simulink model "Traj_track_mec_MAS"  (R2024b)
settings: Solver=ode3  StartTime=0.0  StopTime=300  FixedStep=0.1  RelTol=1e-3
libraries: slpidlib x8
settings Model: Creator=my  LastModifiedBy=my
settings DebuggingCC: AlgebraicLoopMsg=none

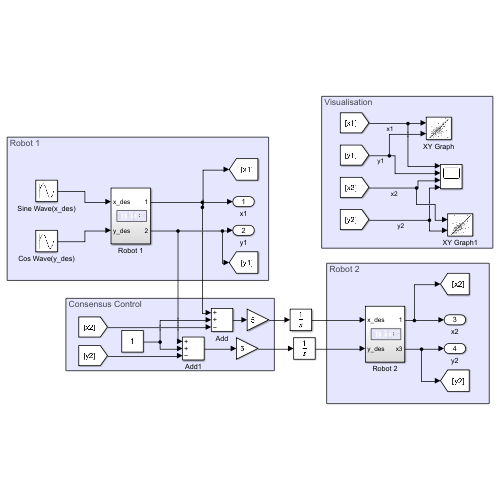
[thumbnail: Simulink's stored preview of the top-level diagram]
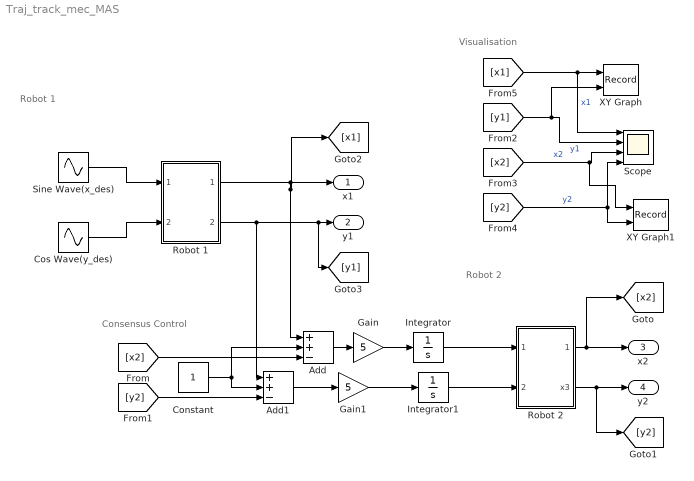
== system Traj_track_mec_MAS ==
  note: Visualisation
  note: Robot 2
  note: Robot 1
  note: Consensus Control
  Add : Sum  Inputs=++-
  Add1 : Sum  Inputs=++-
  Constant : Constant
  Cos Wave(y_des) : Sin  Frequency=0.1  Phase=pi/2  SampleTime=0
  Gain : Gain  Gain=5
  Gain1 : Gain  Gain=5
  Integrator : Integrator
  Integrator1 : Integrator
  Robot 1 : Subsystem
  Robot 2 : Subsystem
  Scope : Scope  NumInputPorts=4
  Sine Wave(x_des) : Sin  Frequency=0.1  SampleTime=0
  XY Graph : Record  FileSettingsInternal="{\"entries\":[{\"content\":{\"excelSettings\":{\"content\":{},\"type\":\"Streamout.ExcelSettings\"}},\"type\":\"Streamout.FileSettingStorage\",\"uuid\":\"\"}],\"packageUris\":[\"http:\\/\\/schema.mathworks.com\\/mf0\\/streamout_blocks\\/R2020a\"],\"version\":\"1.0\"}"  Layout=[1 1]  SignalsInternal="{\"entries\":[{\"content\":{\"signals\":[{\"content\":{\"blockPath\":[],\"dimensions\":[1],\"domain\":\"\",\"lineColor\":\"#a2142f\",\"plots\":[ 1 ],\"port\":1,\"sid\":[\"\"],\"signalID\":1,\"signalName\":\"x1\"},\"type\":\"RecordBlkView.Signal\",\"uuid\":\"\"},{\"content\":{\"blockPath\":[],\"dimensions\":[1],\"domain\":\"\",\"lineColor\":\"#139fff\",\"plots\":[ 1 ],\"port\":2,\"sid\":[\"\"],\"signalID\":2,\"signalName\":\"y1\"},\"type\":\"RecordBlkView.Signal\",\"uuid\":\"\"}]},\"type\":\"RecordBlkView.InputSignals\",\"uuid\":\"\"}],\"packageUris\":[\"http:\\/\\/schema.mathworks.com\\/mf0\\/streamout_blocks\\/R2020a\"],\"version\":\"1.0\"}"  VisualizationBindings="{\"xyplotplugin\":{\"info\":[{\"series\":[{\"bindingParametersList\":[{\"parameter\":\"X-Axis\",\"signalID\":1,\"signalName\":\"x1\"},{\"parameter\":\"Y-Axis\",\"signalID\":2,\"signalName\":\"y1\"}],\"seriesID\":0}],\"subplotID\":1}]}}"  CompatibilityTag=XY
  XY Graph1 : Record  FileSettingsInternal="{\"entries\":[{\"content\":{\"excelSettings\":{\"content\":{},\"type\":\"Streamout.ExcelSettings\"}},\"type\":\"Streamout.FileSettingStorage\",\"uuid\":\"\"}],\"packageUris\":[\"http:\\/\\/schema.mathworks.com\\/mf0\\/streamout_blocks\\/R2020a\"],\"version\":\"1.0\"}"  Layout=[1 1]  SignalsInternal="{\"entries\":[{\"content\":{\"signals\":[{\"content\":{\"blockPath\":[],\"dimensions\":[1],\"domain\":\"\",\"lineColor\":\"#a2142f\",\"plots\":[ 1 ],\"port\":1,\"sid\":[\"\"],\"signalID\":1,\"signalName\":\"x2\"},\"type\":\"RecordBlkView.Signal\",\"uuid\":\"\"},{\"content\":{\"blockPath\":[],\"dimensions\":[1],\"domain\":\"\",\"lineColor\":\"#139fff\",\"plots\":[ 1 ],\"port\":2,\"sid\":[\"\"],\"signalID\":2,\"signalName\":\"y2\"},\"type\":\"RecordBlkView.Signal\",\"uuid\":\"\"}]},\"type\":\"RecordBlkView.InputSignals\",\"uuid\":\"\"}],\"packageUris\":[\"http:\\/\\/schema.mathworks.com\\/mf0\\/streamout_blocks\\/R2020a\"],\"version\":\"1.0\"}"  VisualizationBindings="{\"xyplotplugin\":{\"info\":[{\"series\":[{\"bindingParametersList\":[{\"parameter\":\"X-Axis\",\"signalID\":1,\"signalName\":\"x2\"},{\"parameter\":\"Y-Axis\",\"signalID\":2,\"signalName\":\"y2\"}],\"seriesID\":0}],\"subplotID\":1}]}}"  CompatibilityTag=XY
  x1 : Outport
  y1 : Outport  Port=2
  x2 : Outport  Port=3
  y2 : Outport  Port=4
  wires:
  Sine Wave(x_des)/1 -> Robot 1/1(x_des)
  Cos Wave(y_des)/1 -> Robot 1/2(y_des)
  Robot 1/2(Out2) -> Add1/1, [y1], y1/1
  Robot 2/1(Out1) -> [x2], x2/1
  Robot 2/2(x3) -> [y2], y2/1
  Add/1 -> Gain/1
  Add1/1 -> Gain1/1
  Robot 1/1(Out1) -> [x1], Add/1, x1/1
  [x1] -> XY Graph/1, Scope/1  "x1"
  [y1] -> XY Graph/2, Scope/2  "y1"
  [x2] -> XY Graph1/1, Scope/3  "x2"
  [y2] -> XY Graph1/2, Scope/4  "y2"
  [x2] -> Add/3
  [y2] -> Add1/3
  Constant/1 -> Add/2, Add1/2
  Gain/1 -> Integrator/1
  Integrator/1 -> Robot 2/1(x_des)
  Gain1/1 -> Integrator1/1
  Integrator1/1 -> Robot 2/2(y_des)

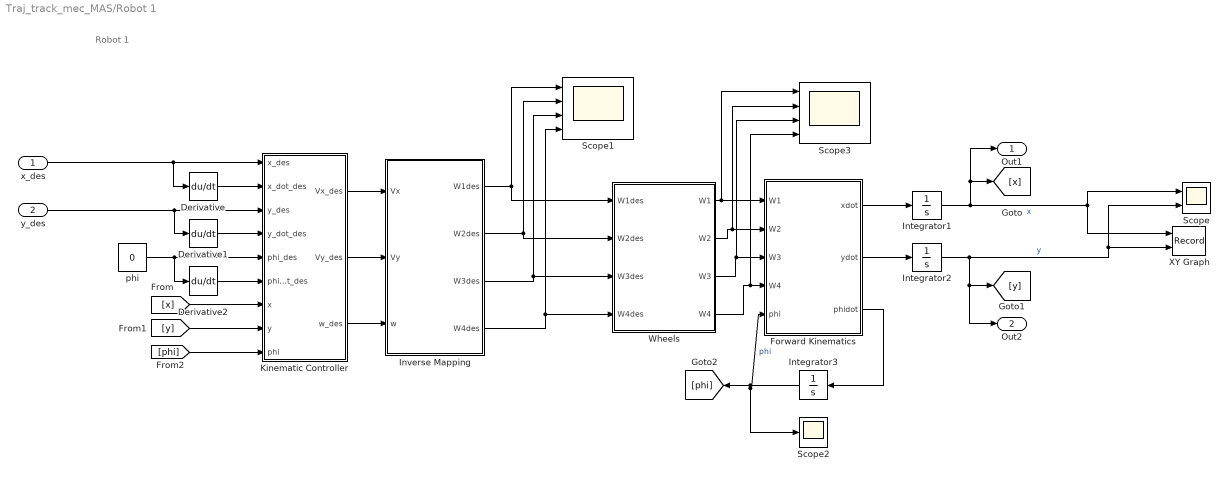
== system Traj_track_mec_MAS/Robot 1 ==
  note: Robot 1
  x_des : Inport
  y_des : Inport  Port=2
  Derivative : Derivative
  Derivative1 : Derivative
  Derivative2 : Derivative
  Forward Kinematics : MATLAB Function  TreatAsAtomicUnit=on
  Integrator1 : Integrator
  Integrator2 : Integrator
  Integrator3 : Integrator
  Inverse Mapping : MATLAB Function  TreatAsAtomicUnit=on
  Kinematic Controller : MATLAB Function  TreatAsAtomicUnit=on
  Scope : Scope  NumInputPorts=2
  Scope1 : Scope  NumInputPorts=4
  Scope2 : Scope
  Scope3 : Scope  NumInputPorts=4
  Wheels : Subsystem
  XY Graph : Record  FileSettingsInternal="{\"entries\":[{\"content\":{\"excelSettings\":{\"content\":{},\"type\":\"Streamout.ExcelSettings\"}},\"type\":\"Streamout.FileSettingStorage\",\"uuid\":\"\"}],\"packageUris\":[\"http:\\/\\/schema.mathworks.com\\/mf0\\/streamout_blocks\\/R2020a\"],\"version\":\"1.0\"}"  Layout=[1 1]  SignalsInternal="{\"entries\":[{\"content\":{\"signals\":[{\"content\":{\"blockPath\":[],\"dimensions\":[1],\"domain\":\"\",\"lineColor\":\"#a2142f\",\"plots\":[ 1 ],\"port\":1,\"sid\":[\"\"],\"signalID\":1,\"signalName\":\"x\"},\"type\":\"RecordBlkView.Signal\",\"uuid\":\"\"},{\"content\":{\"blockPath\":[],\"dimensions\":[1],\"domain\":\"\",\"lineColor\":\"#139fff\",\"plots\":[ 1 ],\"port\":2,\"sid\":[\"\"],\"signalID\":2,\"signalName\":\"y\"},\"type\":\"RecordBlkView.Signal\",\"uuid\":\"\"}]},\"type\":\"RecordBlkView.InputSignals\",\"uuid\":\"\"}],\"packageUris\":[\"http:\\/\\/schema.mathworks.com\\/mf0\\/streamout_blocks\\/R2020a\"],\"version\":\"1.0\"}"  VisualizationBindings="{\"xyplotplugin\":{\"info\":[{\"series\":[{\"bindingParametersList\":[{\"parameter\":\"X-Axis\",\"signalID\":1,\"signalName\":\"x\"},{\"parameter\":\"Y-Axis\",\"signalID\":2,\"signalName\":\"y\"}],\"seriesID\":0}],\"subplotID\":1}]}}"  CompatibilityTag=XY
  phi : Constant  Value=0
  Out1 : Outport
  Out2 : Outport  Port=2
  wires:
  Inverse Mapping/2(W2des) -> Wheels/2(W2des), Scope1/2
  y_des/1 -> Derivative1/1, Kinematic Controller/3(y_des)
  Derivative2/1 -> Kinematic Controller/6(phi_dot_des)
  Wheels/2(W2) -> Scope3/2, Forward Kinematics/2(W2)
  Inverse Mapping/3(W3des) -> Scope1/3, Wheels/3(W3des)
  Forward Kinematics/3(phidot) -> Integrator3/1
  x_des/1 -> Derivative/1, Kinematic Controller/1(x_des)
  Derivative/1 -> Kinematic Controller/2(x_dot_des)
  Integrator3/1 -> [phi], Forward Kinematics/5(phi), Scope2/1  "phi"
  Derivative1/1 -> Kinematic Controller/4(y_dot_des)
  Integrator2/1 -> XY Graph/2, Scope/2, Out2/1, [y]  "y"
  phi/1 -> Kinematic Controller/5(phi_des), Derivative2/1
  Integrator1/1 -> XY Graph/1, Scope/1, Out1/1, [x]  "x"
  Inverse Mapping/4(W4des) -> Scope1/4, Wheels/4(W4des)
  Kinematic Controller/1(Vx_des) -> Inverse Mapping/1(Vx)
  Wheels/1(W1) -> Scope3/1, Forward Kinematics/1(W1)
  Kinematic Controller/3(w_des) -> Inverse Mapping/3(w)
  [x] -> Kinematic Controller/7(x)
  Wheels/4(W4) -> Scope3/4, Forward Kinematics/4(W4)
  Inverse Mapping/1(W1des) -> Wheels/1(W1des), Scope1/1
  Forward Kinematics/1(xdot) -> Integrator1/1
  [y] -> Kinematic Controller/8(y)
  [phi] -> Kinematic Controller/9(phi)
  Wheels/3(W3) -> Scope3/3, Forward Kinematics/3(W3)
  Forward Kinematics/2(ydot) -> Integrator2/1
  Kinematic Controller/2(Vy_des) -> Inverse Mapping/2(Vy)

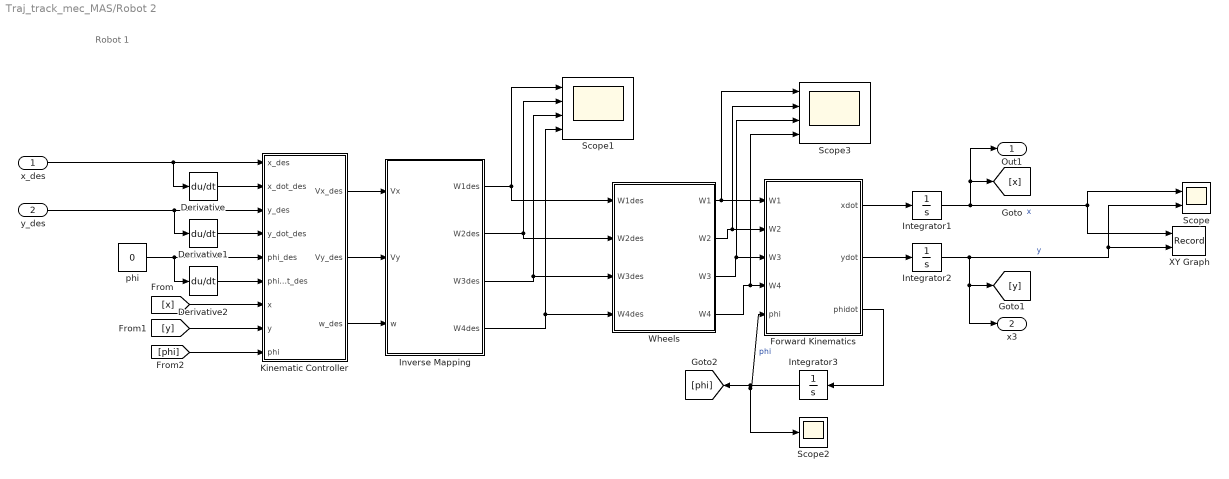
== system Traj_track_mec_MAS/Robot 2 ==
  note: Robot 1
  x_des : Inport
  y_des : Inport  Port=2
  Derivative : Derivative
  Derivative1 : Derivative
  Derivative2 : Derivative
  Forward Kinematics : MATLAB Function  TreatAsAtomicUnit=on
  Integrator1 : Integrator  InitialCondition=2
  Integrator2 : Integrator  InitialCondition=2
  Integrator3 : Integrator
  Inverse Mapping : MATLAB Function  TreatAsAtomicUnit=on
  Kinematic Controller : MATLAB Function  TreatAsAtomicUnit=on
  Scope : Scope  NumInputPorts=2
  Scope1 : Scope  NumInputPorts=4
  Scope2 : Scope
  Scope3 : Scope  NumInputPorts=4
  Wheels : Subsystem
  XY Graph : Record  FileSettingsInternal="{\"entries\":[{\"content\":{\"excelSettings\":{\"content\":{},\"type\":\"Streamout.ExcelSettings\"}},\"type\":\"Streamout.FileSettingStorage\",\"uuid\":\"\"}],\"packageUris\":[\"http:\\/\\/schema.mathworks.com\\/mf0\\/streamout_blocks\\/R2020a\"],\"version\":\"1.0\"}"  Layout=[1 1]  SignalsInternal="{\"entries\":[{\"content\":{\"signals\":[{\"content\":{\"blockPath\":[],\"dimensions\":[1],\"domain\":\"\",\"lineColor\":\"#a2142f\",\"plots\":[ 1 ],\"port\":1,\"sid\":[\"\"],\"signalID\":1,\"signalName\":\"x\"},\"type\":\"RecordBlkView.Signal\",\"uuid\":\"\"},{\"content\":{\"blockPath\":[],\"dimensions\":[1],\"domain\":\"\",\"lineColor\":\"#139fff\",\"plots\":[ 1 ],\"port\":2,\"sid\":[\"\"],\"signalID\":2,\"signalName\":\"y\"},\"type\":\"RecordBlkView.Signal\",\"uuid\":\"\"}]},\"type\":\"RecordBlkView.InputSignals\",\"uuid\":\"\"}],\"packageUris\":[\"http:\\/\\/schema.mathworks.com\\/mf0\\/streamout_blocks\\/R2020a\"],\"version\":\"1.0\"}"  VisualizationBindings="{\"xyplotplugin\":{\"info\":[{\"series\":[{\"bindingParametersList\":[{\"parameter\":\"X-Axis\",\"signalID\":1,\"signalName\":\"x\"},{\"parameter\":\"Y-Axis\",\"signalID\":2,\"signalName\":\"y\"}],\"seriesID\":0}],\"subplotID\":1}]}}"  CompatibilityTag=XY
  phi : Constant  Value=0
  Out1 : Outport
  x3 : Outport  Port=2
  wires:
  Inverse Mapping/2(W2des) -> Wheels/2(W2des), Scope1/2
  y_des/1 -> Derivative1/1, Kinematic Controller/3(y_des)
  Derivative2/1 -> Kinematic Controller/6(phi_dot_des)
  Wheels/2(W2) -> Scope3/2, Forward Kinematics/2(W2)
  Inverse Mapping/3(W3des) -> Scope1/3, Wheels/3(W3des)
  Forward Kinematics/3(phidot) -> Integrator3/1
  x_des/1 -> Derivative/1, Kinematic Controller/1(x_des)
  Derivative/1 -> Kinematic Controller/2(x_dot_des)
  Integrator3/1 -> [phi], Forward Kinematics/5(phi), Scope2/1  "phi"
  Derivative1/1 -> Kinematic Controller/4(y_dot_des)
  Integrator2/1 -> XY Graph/2, Scope/2, x3/1, [y]  "y"
  phi/1 -> Kinematic Controller/5(phi_des), Derivative2/1
  Integrator1/1 -> XY Graph/1, Scope/1, Out1/1, [x]  "x"
  Inverse Mapping/4(W4des) -> Scope1/4, Wheels/4(W4des)
  Kinematic Controller/1(Vx_des) -> Inverse Mapping/1(Vx)
  Wheels/1(W1) -> Scope3/1, Forward Kinematics/1(W1)
  Kinematic Controller/3(w_des) -> Inverse Mapping/3(w)
  [x] -> Kinematic Controller/7(x)
  Wheels/4(W4) -> Scope3/4, Forward Kinematics/4(W4)
  Inverse Mapping/1(W1des) -> Wheels/1(W1des), Scope1/1
  Forward Kinematics/1(xdot) -> Integrator1/1
  [y] -> Kinematic Controller/8(y)
  [phi] -> Kinematic Controller/9(phi)
  Wheels/3(W3) -> Scope3/3, Forward Kinematics/3(W3)
  Forward Kinematics/2(ydot) -> Integrator2/1
  Kinematic Controller/2(Vy_des) -> Inverse Mapping/2(Vy)

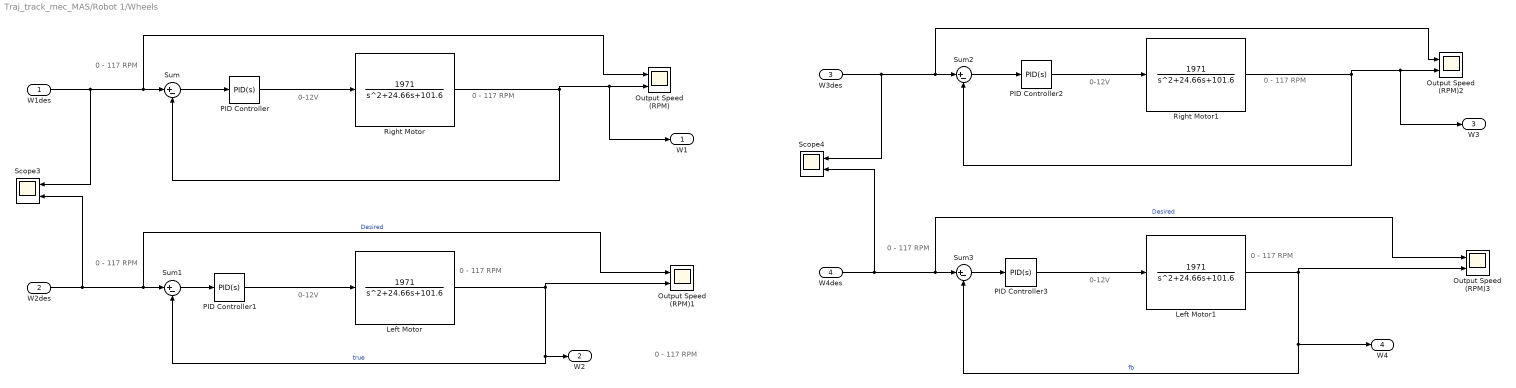
== system Traj_track_mec_MAS/Robot 1/Wheels ==
  note: 0 - 117 RPM
  note: 0-12V
  note: 0 - 117 RPM
  note: 0 - 117 RPM
  note: 0-12V
  note: 0 - 117 RPM
  note: 0 - 117 RPM
  note: 0-12V
  note: 0 - 117 RPM
  note: 0 - 117 RPM
  note: 0-12V
  note: 0 - 117 RPM
  W1des : Inport
  W2des : Inport  Port=2
  W3des : Inport  Port=3
  W4des : Inport  Port=4
  Left Motor : TransferFcn  Numerator=1971  Denominator=[1 24.66 101.6]
  Left Motor1 : TransferFcn  Numerator=1971  Denominator=[1 24.66 101.6]
  Output Speed (RPM){,1..3} (4 alike) : Scope  NumInputPorts=2
  PID Controller{,1..3} (4 alike) : slpidlib/PID Controller  Controller=PID  Form=Parallel  TimeDomain=Continuous-time  UseExternalTs=off  SampleTime=-1  IntegratorMethod=Forward Euler  FilterMethod=Forward Euler  ControllerParametersSource=internal  P=3  I=0  UseKiTs=off  D=0  UseExternalDerivativeSource=off  N=100  UseFilter=on  TunerSelectOption=Transfer Function Based (PID Tuner App)  InitialConditionSource=internal  InitialConditionForIntegrator=0  InitialConditionForFilter=0  DifferentiatorICPrevScaledInput=0  ExternalReset=none  TrackingMode=off  Kt=1  LimitOutput=on  SatLimitsSource=internal  UpperSaturationLimit=12  LowerSaturationLimit=-12  LinearizeAsGain=on  AntiWindupMode=none  Kb=1  LimitIntegrator=off  UpperIntegratorSaturationLimit=inf  LowerIntegratorSaturationLimit=-inf  POutMin=[]  POutMax=[]  IOutMin=[]  IOutMax=[]  DOutMin=[]  DOutMax=[]  NOutMin=[]  NOutMax=[]  SumOutMin=[]  SumOutMax=[]  SaturationOutMin=[]  SaturationOutMax=[]  PParamMin=[]  PParamMax=[]  IParamMin=[]  IParamMax=[]  DParamMin=[]  DParamMax=[]  NParamMin=[]  NParamMax=[]  KbParamMin=[]  KbParamMax=[]  KtParamMin=[]  KtParamMax=[]  KbOutMin=[]  KbOutMax=[]  KtOutMin=[]  KtOutMax=[]  IntegratorOutMin=[]  IntegratorOutMax=[]  FilterOutMin=[]  FilterOutMax=[]  SumI1OutMin=[]  SumI1OutMax=[]  SumI2OutMin=[]  SumI2OutMax=[]  SumI3OutMin=[]  SumI3OutMax=[]  SumI4OutMin=[]  SumI4OutMax=[]  SumDOutMin=[]  SumDOutMax=[]  DifferentiatorOutMin=[]  DifferentiatorOutMax=[]  FilterDiffOutCoefMin=[]  FilterDiffOutCoefMax=[]  ReciprocalOutMin=[]  ReciprocalOutMax=[]  SumDenOutMin=[]  SumDenOutMax=[]  SumNumOutMin=[]  SumNumOutMax=[]  DivideOutMin=[]  DivideOutMax=[]  UdiffTsProdOutMin=[]  UdiffTsProdOutMax=[]  NTsProdOutMin=[]  NTsProdOutMax=[]  UintegralTsProdOutMin=[]  UintegralTsProdOutMax=[]  UngainTsProdOutMin=[]  UngainTsProdOutMax=[]  ClampingZeroOutDataTypeStr=Inherit: Inherit via back propagation  ClampingZeroOutMin=[]  ClampingZeroOutMax=[]  FilterDenConstantOutDataTypeStr=Inherit: Inherit via back propagation  FilterDenConstantOutMin=[]  FilterDenConstantOutMax=[]  PCopyOutDataTypeStr=Inherit: Inherit via back propagation  PCopyOutMin=[]  PCopyOutMax=[]  NCopyOutDataTypeStr=Inherit: Inherit via back propagation  NCopyOutMin=[]  NCopyOutMax=[]  IntegratorContinuousStateAttributes=''  IntegratorStateMustResolveToSignalObject=off  IntegratorRTWStateStorageClass=Auto  FilterContinuousStateAttributes=''  FilterStateMustResolveToSignalObject=off  FilterRTWStateStorageClass=Auto  ParallelPVariant=InternalParameters  IdealPVariant=Disabled  IVariant=InternalParameters  DVariant=InternalParameters  IntegratorVariant=Continuous  SatVariant=Enabled  AWVariant=Passthrough  PCopyVariant=Disabled  TRVariant=Disabled  FdbkBlocksVariant=Forward  IdealPFdbkVariant=Disabled  SatFdbkVariant=Disabled  DerivativeFilterVariant=ContFilter  NVariant=InternalParameters  NCopyVariant=Disabled  FilterICVariant=InternalICsFilter  IntegratorICVariant=InternalICs  ExternalResetVariant=Disabled  TRSumVariant=Passthrough  SumFdbkVariant=Disabled  SumVariant=Sum_PID  TsampFilterVariant=InternalTs  TsampNgainVariant=Passthrough  TsampIntegralVariant=Disabled_SignalSpec  ExternalSaturationOutDataTypeStr=Inherit: Same as second input  DerivativeSourceVariant=ErrorSignal  PreIntVariant=InternalPreInt
  Right Motor : TransferFcn  Numerator=1971  Denominator=[1 24.66 101.6]
  Right Motor1 : TransferFcn  Numerator=1971  Denominator=[1 24.66 101.6]
  Scope3 : Scope  NumInputPorts=2
  Scope4 : Scope  NumInputPorts=2
  Sum{,1..3} (4 alike) : Sum  Inputs=|+-
  W1 : Outport
  W2 : Outport  Port=2
  W3 : Outport  Port=3
  W4 : Outport  Port=4
  wires:
  W2des/1 -> Scope3/2, Output Speed (RPM)1/1, Sum1/1  "Desired"
  Right Motor/1 -> Sum/2, W1/1, Output Speed (RPM)/2
  PID Controller/1 -> Right Motor/1
  Sum/1 -> PID Controller/1
  Sum1/1 -> PID Controller1/1
  W1des/1 -> Scope3/1, Output Speed (RPM)/1, Sum/1
  Left Motor/1 -> Output Speed (RPM)1/2, W2/1, Sum1/2  "true"
  PID Controller1/1 -> Left Motor/1
  PID Controller3/1 -> Left Motor1/1
  W3des/1 -> Sum2/1, Output Speed (RPM)2/1, Scope4/1
  Sum3/1 -> PID Controller3/1
  Sum2/1 -> PID Controller2/1
  PID Controller2/1 -> Right Motor1/1
  Right Motor1/1 -> Output Speed (RPM)2/2, W3/1, Sum2/2
  W4des/1 -> Output Speed (RPM)3/1, Sum3/1, Scope4/2  "Desired"
  Left Motor1/1 -> Output Speed (RPM)3/2, Sum3/2, W4/1  "fb"

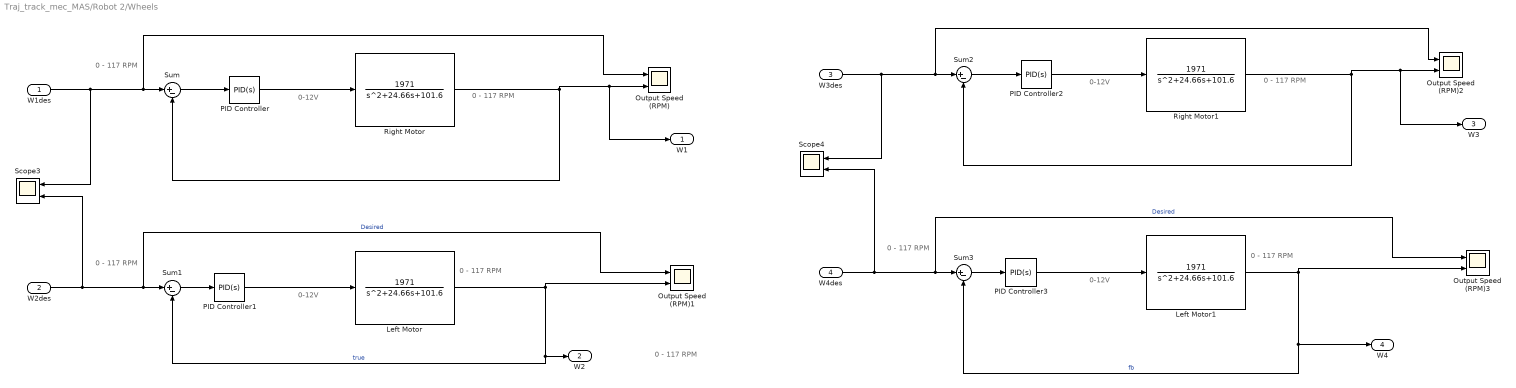
== system Traj_track_mec_MAS/Robot 2/Wheels ==
  note: 0 - 117 RPM
  note: 0-12V
  note: 0 - 117 RPM
  note: 0 - 117 RPM
  note: 0-12V
  note: 0 - 117 RPM
  note: 0 - 117 RPM
  note: 0-12V
  note: 0 - 117 RPM
  note: 0 - 117 RPM
  note: 0-12V
  note: 0 - 117 RPM
  W1des : Inport
  W2des : Inport  Port=2
  W3des : Inport  Port=3
  W4des : Inport  Port=4
  Left Motor : TransferFcn  Numerator=1971  Denominator=[1 24.66 101.6]
  Left Motor1 : TransferFcn  Numerator=1971  Denominator=[1 24.66 101.6]
  Output Speed (RPM){,1..3} (4 alike) : Scope  NumInputPorts=2
  PID Controller{,1..3} (4 alike) : slpidlib/PID Controller  Controller=PID  Form=Parallel  TimeDomain=Continuous-time  UseExternalTs=off  SampleTime=-1  IntegratorMethod=Forward Euler  FilterMethod=Forward Euler  ControllerParametersSource=internal  P=3  I=0  UseKiTs=off  D=0  UseExternalDerivativeSource=off  N=100  UseFilter=on  TunerSelectOption=Transfer Function Based (PID Tuner App)  InitialConditionSource=internal  InitialConditionForIntegrator=0  InitialConditionForFilter=0  DifferentiatorICPrevScaledInput=0  ExternalReset=none  TrackingMode=off  Kt=1  LimitOutput=on  SatLimitsSource=internal  UpperSaturationLimit=12  LowerSaturationLimit=-12  LinearizeAsGain=on  AntiWindupMode=none  Kb=1  LimitIntegrator=off  UpperIntegratorSaturationLimit=inf  LowerIntegratorSaturationLimit=-inf  POutMin=[]  POutMax=[]  IOutMin=[]  IOutMax=[]  DOutMin=[]  DOutMax=[]  NOutMin=[]  NOutMax=[]  SumOutMin=[]  SumOutMax=[]  SaturationOutMin=[]  SaturationOutMax=[]  PParamMin=[]  PParamMax=[]  IParamMin=[]  IParamMax=[]  DParamMin=[]  DParamMax=[]  NParamMin=[]  NParamMax=[]  KbParamMin=[]  KbParamMax=[]  KtParamMin=[]  KtParamMax=[]  KbOutMin=[]  KbOutMax=[]  KtOutMin=[]  KtOutMax=[]  IntegratorOutMin=[]  IntegratorOutMax=[]  FilterOutMin=[]  FilterOutMax=[]  SumI1OutMin=[]  SumI1OutMax=[]  SumI2OutMin=[]  SumI2OutMax=[]  SumI3OutMin=[]  SumI3OutMax=[]  SumI4OutMin=[]  SumI4OutMax=[]  SumDOutMin=[]  SumDOutMax=[]  DifferentiatorOutMin=[]  DifferentiatorOutMax=[]  FilterDiffOutCoefMin=[]  FilterDiffOutCoefMax=[]  ReciprocalOutMin=[]  ReciprocalOutMax=[]  SumDenOutMin=[]  SumDenOutMax=[]  SumNumOutMin=[]  SumNumOutMax=[]  DivideOutMin=[]  DivideOutMax=[]  UdiffTsProdOutMin=[]  UdiffTsProdOutMax=[]  NTsProdOutMin=[]  NTsProdOutMax=[]  UintegralTsProdOutMin=[]  UintegralTsProdOutMax=[]  UngainTsProdOutMin=[]  UngainTsProdOutMax=[]  ClampingZeroOutDataTypeStr=Inherit: Inherit via back propagation  ClampingZeroOutMin=[]  ClampingZeroOutMax=[]  FilterDenConstantOutDataTypeStr=Inherit: Inherit via back propagation  FilterDenConstantOutMin=[]  FilterDenConstantOutMax=[]  PCopyOutDataTypeStr=Inherit: Inherit via back propagation  PCopyOutMin=[]  PCopyOutMax=[]  NCopyOutDataTypeStr=Inherit: Inherit via back propagation  NCopyOutMin=[]  NCopyOutMax=[]  IntegratorContinuousStateAttributes=''  IntegratorStateMustResolveToSignalObject=off  IntegratorRTWStateStorageClass=Auto  FilterContinuousStateAttributes=''  FilterStateMustResolveToSignalObject=off  FilterRTWStateStorageClass=Auto  ParallelPVariant=InternalParameters  IdealPVariant=Disabled  IVariant=InternalParameters  DVariant=InternalParameters  IntegratorVariant=Continuous  SatVariant=Enabled  AWVariant=Passthrough  PCopyVariant=Disabled  TRVariant=Disabled  FdbkBlocksVariant=Forward  IdealPFdbkVariant=Disabled  SatFdbkVariant=Disabled  DerivativeFilterVariant=ContFilter  NVariant=InternalParameters  NCopyVariant=Disabled  FilterICVariant=InternalICsFilter  IntegratorICVariant=InternalICs  ExternalResetVariant=Disabled  TRSumVariant=Passthrough  SumFdbkVariant=Disabled  SumVariant=Sum_PID  TsampFilterVariant=InternalTs  TsampNgainVariant=Passthrough  TsampIntegralVariant=Disabled_SignalSpec  ExternalSaturationOutDataTypeStr=Inherit: Same as second input  DerivativeSourceVariant=ErrorSignal  PreIntVariant=InternalPreInt
  Right Motor : TransferFcn  Numerator=1971  Denominator=[1 24.66 101.6]
  Right Motor1 : TransferFcn  Numerator=1971  Denominator=[1 24.66 101.6]
  Scope3 : Scope  NumInputPorts=2
  Scope4 : Scope  NumInputPorts=2
  Sum{,1..3} (4 alike) : Sum  Inputs=|+-
  W1 : Outport
  W2 : Outport  Port=2
  W3 : Outport  Port=3
  W4 : Outport  Port=4
  wires:
  W2des/1 -> Scope3/2, Output Speed (RPM)1/1, Sum1/1  "Desired"
  Right Motor/1 -> Sum/2, W1/1, Output Speed (RPM)/2
  PID Controller/1 -> Right Motor/1
  Sum/1 -> PID Controller/1
  Sum1/1 -> PID Controller1/1
  W1des/1 -> Scope3/1, Output Speed (RPM)/1, Sum/1
  Left Motor/1 -> Output Speed (RPM)1/2, W2/1, Sum1/2  "true"
  PID Controller1/1 -> Left Motor/1
  PID Controller3/1 -> Left Motor1/1
  W3des/1 -> Sum2/1, Output Speed (RPM)2/1, Scope4/1
  Sum3/1 -> PID Controller3/1
  Sum2/1 -> PID Controller2/1
  PID Controller2/1 -> Right Motor1/1
  Right Motor1/1 -> Output Speed (RPM)2/2, W3/1, Sum2/2
  W4des/1 -> Output Speed (RPM)3/1, Sum3/1, Scope4/2  "Desired"
  Left Motor1/1 -> Output Speed (RPM)3/2, Sum3/2, W4/1  "fb"

== matlab function Traj_track_mec_MAS/Robot 1/Inverse Mapping ==
  data: Vx input; W1des output; W2des output; W3des output; W4des output; Vy input; w input
function [W1des,W2des,W3des,W4des] = fcn(Vx,Vy,w)

r = 0.04;
Lx = 0.09;
Ly = 0.095;
%% Define matrix M
M = (1/r)*[1,-1,-(Lx+Ly); 1,1,Lx+Ly;1,1,-(Lx+Ly);1,-1,(Lx+Ly)];

Wheel_speeds = M*[Vx;Vy;w];

W1des = Wheel_speeds(1);
W2des =  Wheel_speeds(2);
W3des = Wheel_speeds(3);
W4des =  Wheel_speeds(4);

%convert rad/sec to RPM

W1des = (60/(2*pi))*W1des;
W2des = (60/(2*pi))*W2des;
W3des = (60/(2*pi))*W3des;
W4des = (60/(2*pi))*W4des;

== matlab function Traj_track_mec_MAS/Robot 1/Forward Kinematics ==
  data: W1 input; xdot output; W2 input; W3 input; W4 input; ydot output; phidot output; phi input
function [xdot,ydot,phidot] = fcn(W1,W2,W3,W4,phi)

r = 0.04;
Lx = 0.09;
Ly = 0.095;

%convert RW,LW from RPM to rad/sec.

W1 = W1*(2*pi/60);
W2 = W2*(2*pi/60);
W3 = W3*(2*pi/60);
W4 = W4*(2*pi/60);

Vx = r*(W1 + W2 + W3 + W4)/4;
Vy = r*(-W1 + W2 + W3 - W4)/4;
w = r*(-W1 + W2 -W3 + W4)/(4*(Lx+Ly));


xdot = Vx*cos(phi) - Vy*sin(phi);
ydot = Vx*sin(phi) + Vy*cos(phi);
phidot = w;

== matlab function Traj_track_mec_MAS/Robot 1/Kinematic Controller ==
  data: x_des input; x_dot_des input; Vx_des output; y_des input; y_dot_des input; phi_des input; phi_dot_des input; x input; y input; Vy_des output; w_des output; phi input
function [Vx_des,Vy_des,w_des] = fcn(x_des,x_dot_des,y_des,y_dot_des,phi_des, phi_dot_des, x,y,phi)

T = [cos(phi),-sin(phi),0;
     sin(phi),cos(phi),0;
     0,0,1];

kx = 3;
ky = 3;
kphi = 1;

V = inv(T)*[x_dot_des + kx* tanh(x_des - x);
            y_dot_des + ky* tanh(y_des - y);
            phi_dot_des + kphi* tanh(phi_des - phi)];

Vx_des = V(1);
Vy_des = V(2);
w_des = V(3);

== matlab function Traj_track_mec_MAS/Robot 2/Forward Kinematics ==
  data: W1 input; xdot output; W2 input; W3 input; W4 input; ydot output; phidot output; phi input
function [xdot,ydot,phidot] = fcn(W1,W2,W3,W4,phi)

r = 0.04;
Lx = 0.09;
Ly = 0.095;

%convert RW,LW from RPM to rad/sec.

W1 = W1*(2*pi/60);
W2 = W2*(2*pi/60);
W3 = W3*(2*pi/60);
W4 = W4*(2*pi/60);

Vx = r*(W1 + W2 + W3 + W4)/4;
Vy = r*(-W1 + W2 + W3 - W4)/4;
w = r*(-W1 + W2 -W3 + W4)/(4*(Lx+Ly));


xdot = Vx*cos(phi) - Vy*sin(phi);
ydot = Vx*sin(phi) + Vy*cos(phi);
phidot = w;

== matlab function Traj_track_mec_MAS/Robot 2/Inverse Mapping ==
  data: Vx input; W1des output; W2des output; W3des output; W4des output; Vy input; w input
function [W1des,W2des,W3des,W4des] = fcn(Vx,Vy,w)

r = 0.04;
Lx = 0.09;
Ly = 0.095;
%% Define matrix M
M = (1/r)*[1,-1,-(Lx+Ly); 1,1,Lx+Ly;1,1,-(Lx+Ly);1,-1,(Lx+Ly)];

Wheel_speeds = M*[Vx;Vy;w];

W1des = Wheel_speeds(1);
W2des =  Wheel_speeds(2);
W3des = Wheel_speeds(3);
W4des =  Wheel_speeds(4);

%convert rad/sec to RPM

W1des = (60/(2*pi))*W1des;
W2des = (60/(2*pi))*W2des;
W3des = (60/(2*pi))*W3des;
W4des = (60/(2*pi))*W4des;

== matlab function Traj_track_mec_MAS/Robot 2/Kinematic Controller ==
  data: x_des input; x_dot_des input; Vx_des output; y_des input; y_dot_des input; phi_des input; phi_dot_des input; x input; y input; Vy_des output; w_des output; phi input
function [Vx_des,Vy_des,w_des] = fcn(x_des,x_dot_des,y_des,y_dot_des,phi_des, phi_dot_des, x,y,phi)

T = [cos(phi),-sin(phi),0;
     sin(phi),cos(phi),0;
     0,0,1];

kx = 3;
ky = 3;
kphi = 1;

V = inv(T)*[x_dot_des + kx* tanh(x_des - x);
            y_dot_des + ky* tanh(y_des - y);
            phi_dot_des + kphi* tanh(phi_des - phi)];

Vx_des = V(1);
Vy_des = V(2);
w_des = V(3);
